simulink model "TRNG_test01"  (R2020a)
settings: Solver=VariableStepAuto  StartTime=0.0  StopTime=100.0  RelTol=1e-3
undefined symbols (not defined in the file): AXI4, Lite
libraries: xbsIndex_r4 x185
settings Model: Creator=ringl  LastModifiedBy=ringl

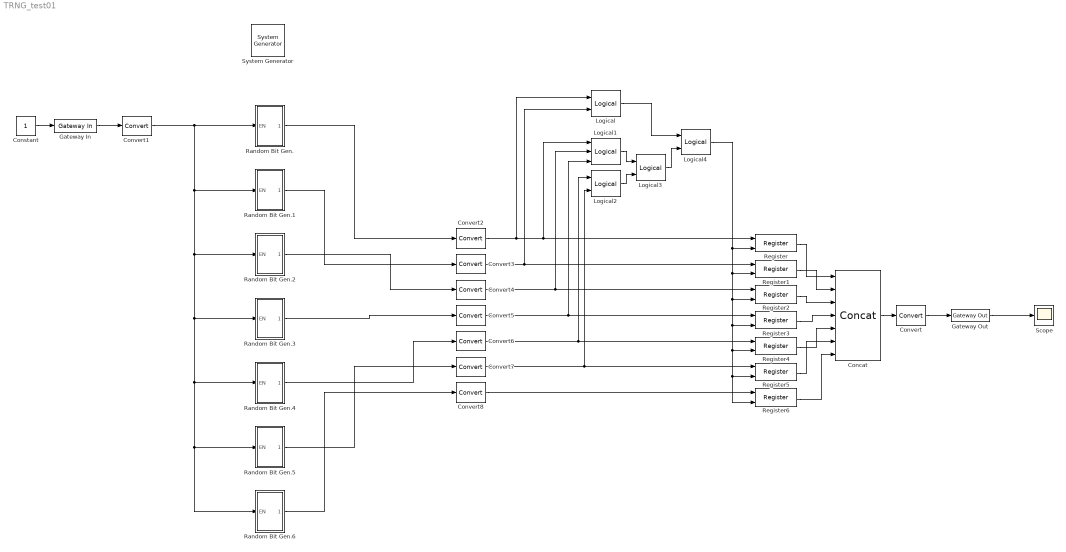
== system TRNG_test01 ==
  " System Generator" : xbsIndex_r4/ System Generator  Tag=genX  xilinxfamily=zynq  part=xc7z020  speed=-1  package=clg400  synthesis_tool=Vivado  clock_wrapper=Clock Enables  directory=./netlist  proj_type=Vivado  Synth_file=Vivado Synthesis Defaults  Impl_file=Vivado Implementation Defaults  testbench=off  simulink_period=1  sysclk_period=10  dcm_input_clock_period=10  incr_netlist=off  trim_vbits=Everywhere in SubSystem  dbl_ovrd=According to Block Masks  core_generation=According to Block Masks  run_coregen=off  deprecated_control=off  eval_field=0  block_type=sysgen
  Concat : xbsIndex_r4/Concat  num_inputs=7  dbl_ovrd=off  block_type=concat
  Constant : Constant
  Convert : xbsIndex_r4/Convert  gui_display_data_type=Fixed-point  arith_type="Signed  (2's comp)"  n_bits=32  bin_pt=0  float_type=Single  exp_bits=8  fraction_bits=24  quantization=Truncate  overflow=Wrap  en=off  latency=1  pipeline=off  dbl_ovrd=off  block_type=convert
  Convert1 : xbsIndex_r4/Convert  gui_display_data_type=Fixed-point  arith_type="Signed  (2's comp)"  n_bits=1  bin_pt=0  float_type=Single  exp_bits=8  fraction_bits=24  quantization=Truncate  overflow=Wrap  en=off  latency=1  pipeline=off  dbl_ovrd=off  block_type=convert
  Convert{2..8} (7 alike) : xbsIndex_r4/Convert  gui_display_data_type=Fixed-point  arith_type=Unsigned  n_bits=1  bin_pt=0  float_type=Single  exp_bits=8  fraction_bits=24  quantization=Truncate  overflow=Wrap  en=off  latency=1  pipeline=off  dbl_ovrd=off  block_type=convert
  Gateway In : xbsIndex_r4/Gateway In  gui_display_data_type=Fixed-point  arith_type="Signed  (2's comp)"  n_bits=32  bin_pt=0  preci_type=Single  exp_width=8  frac_width=24  rows=1  columns=1  quantization="Round  (unbiased: +/- Inf)"  overflow=Saturate  period=1  UseAsADC=off  ADCChannel='1'  interface=AXI4-Lite  automatic_assignment=on  address_offset=hex2dec('00')  intf_name=''  intf_description=''  default_value=0  timing_constraint=None  locs_specified=off  LOCs={}  io_standard={}  inherit_from_input=off  hdl_port=on  dbl_ovrd=off  block_type=gatewayin
  Gateway Out : xbsIndex_r4/Gateway Out  inherit_from_input=off  hdl_port=on  rows=1  columns=1  UseAsDAC=off  DACChannel='1'  interface=AXI4-Lite  automatic_assignment=on  address_offset=hex2dec('00')  intf_name=''  intf_description=''  timing_constraint=None  locs_specified=off  LOCs={}  io_standard={}  block_type=gatewayout
  Logical : xbsIndex_r4/Logical  logical_function=AND  inputs=2  en=off  latency=1  precision=Full  arith_type=Unsigned  n_bits=16  bin_pt=0  align_bp=on  dbl_ovrd=off  block_type=logical
  Logical1 : xbsIndex_r4/Logical  logical_function=AND  inputs=3  en=off  latency=1  precision=Full  arith_type=Unsigned  n_bits=16  bin_pt=0  align_bp=on  dbl_ovrd=off  block_type=logical
  Logical2 : xbsIndex_r4/Logical  logical_function=OR  inputs=2  en=off  latency=1  precision=Full  arith_type=Unsigned  n_bits=16  bin_pt=0  align_bp=on  dbl_ovrd=off  block_type=logical
  Logical3 : xbsIndex_r4/Logical  logical_function=AND  inputs=2  en=off  latency=1  precision=Full  arith_type=Unsigned  n_bits=16  bin_pt=0  align_bp=on  dbl_ovrd=off  block_type=logical
  Logical4 : xbsIndex_r4/Logical  logical_function=NOR  inputs=2  en=off  latency=1  precision=Full  arith_type=Unsigned  n_bits=16  bin_pt=0  align_bp=on  dbl_ovrd=off  block_type=logical
  Random Bit Gen. : Subsystem
  Random Bit Gen.1 : Subsystem
  Random Bit Gen.2 : Subsystem
  Random Bit Gen.3 : Subsystem
  Random Bit Gen.4 : Subsystem
  Random Bit Gen.5 : Subsystem
  Random Bit Gen.6 : Subsystem
  Register{,1..6} (7 alike) : xbsIndex_r4/Register  init=0  rst=off  en=on  dbl_ovrd=off  block_type=register
  Scope : Scope
  wires:
  Constant/1 -> Gateway In/1
  Gateway In/1 -> Convert1/1
  Gateway Out/1 -> Scope/1
  Convert/1 -> Gateway Out/1
  Convert1/1 -> Random Bit Gen.2/1(EN), Random Bit Gen.3/1(EN), Random Bit Gen.4/1(EN), Random Bit Gen.5/1(EN), Random Bit Gen.6/1(EN), Random Bit Gen.1/1(EN), Random Bit Gen./1(EN)
  Random Bit Gen./1(OUT) -> Convert2/1
  Concat/1 -> Convert/1
  Convert2/1 -> Logical/1, Logical1/1, Register/1
  Random Bit Gen.1/1(OUT) -> Convert3/1
  Random Bit Gen.2/1(OUT) -> Convert4/1
  Random Bit Gen.3/1(OUT) -> Convert5/1
  Random Bit Gen.4/1(OUT) -> Convert6/1
  Random Bit Gen.5/1(OUT) -> Convert7/1
  Random Bit Gen.6/1(OUT) -> Convert8/1
  Register3/1 -> Concat/4
  Register4/1 -> Concat/5
  Register5/1 -> Concat/6
  Register6/1 -> Concat/7
  Register2/1 -> Concat/3
  Register1/1 -> Concat/2
  Register/1 -> Concat/1
  Convert3/1 -> Logical/2, Register1/1
  Convert4/1 -> Logical1/2, Register2/1
  Convert5/1 -> Logical1/3, Register3/1
  Convert6/1 -> Logical2/1, Register4/1
  Convert7/1 -> Logical2/2, Register5/1
  Convert8/1 -> Register6/1
  Logical2/1 -> Logical3/2
  Logical1/1 -> Logical3/1
  Logical3/1 -> Logical4/2
  Logical/1 -> Logical4/1
  Logical4/1 -> Register/2, Register1/2, Register2/2, Register3/2, Register4/2, Register5/2, Register6/2

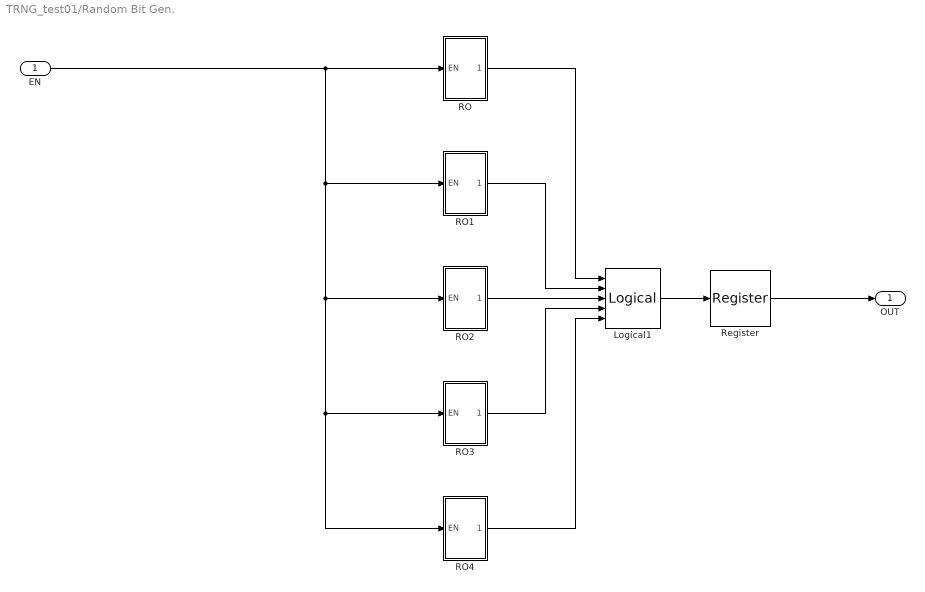
== system TRNG_test01/Random Bit Gen. ==
  EN : Inport
  Logical1 : xbsIndex_r4/Logical  logical_function=XOR  inputs=5  en=off  latency=1  precision=Full  arith_type=Unsigned  n_bits=16  bin_pt=0  align_bp=on  dbl_ovrd=off  block_type=logical
  RO : Subsystem
  RO1 : Subsystem
  RO2 : Subsystem
  RO3 : Subsystem
  RO4 : Subsystem
  Register : xbsIndex_r4/Register  init=0  rst=off  en=off  dbl_ovrd=off  block_type=register
  OUT : Outport
  wires:
  Logical1/1 -> Register/1
  EN/1 -> RO/1(EN), RO1/1(EN), RO2/1(EN), RO4/1(EN), RO3/1(EN)
  RO1/1(OUT) -> Logical1/2
  RO2/1(OUT) -> Logical1/3
  RO/1(OUT) -> Logical1/1
  RO4/1(OUT) -> Logical1/5
  RO3/1(OUT) -> Logical1/4
  Register/1 -> OUT/1

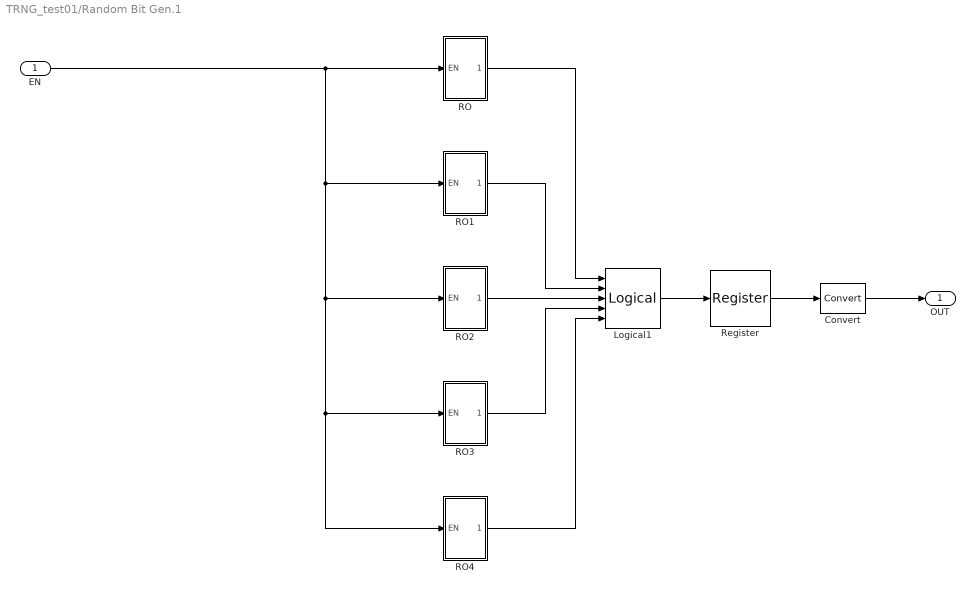
== system TRNG_test01/Random Bit Gen.1 ==
  EN : Inport
  Convert : xbsIndex_r4/Convert  gui_display_data_type=Fixed-point  arith_type="Signed  (2's comp)"  n_bits=1  bin_pt=0  float_type=Single  exp_bits=8  fraction_bits=24  quantization=Truncate  overflow=Wrap  en=off  latency=1  pipeline=off  dbl_ovrd=off  block_type=convert
  Logical1 : xbsIndex_r4/Logical  logical_function=XOR  inputs=5  en=off  latency=1  precision=Full  arith_type=Unsigned  n_bits=16  bin_pt=0  align_bp=on  dbl_ovrd=off  block_type=logical
  RO : Subsystem
  RO1 : Subsystem
  RO2 : Subsystem
  RO3 : Subsystem
  RO4 : Subsystem
  Register : xbsIndex_r4/Register  init=0  rst=off  en=off  dbl_ovrd=off  block_type=register
  OUT : Outport
  wires:
  Logical1/1 -> Register/1
  EN/1 -> RO/1(EN), RO1/1(EN), RO2/1(EN), RO4/1(EN), RO3/1(EN)
  RO1/1(OUT) -> Logical1/2
  RO2/1(OUT) -> Logical1/3
  RO/1(OUT) -> Logical1/1
  RO4/1(OUT) -> Logical1/5
  RO3/1(OUT) -> Logical1/4
  Convert/1 -> OUT/1
  Register/1 -> Convert/1

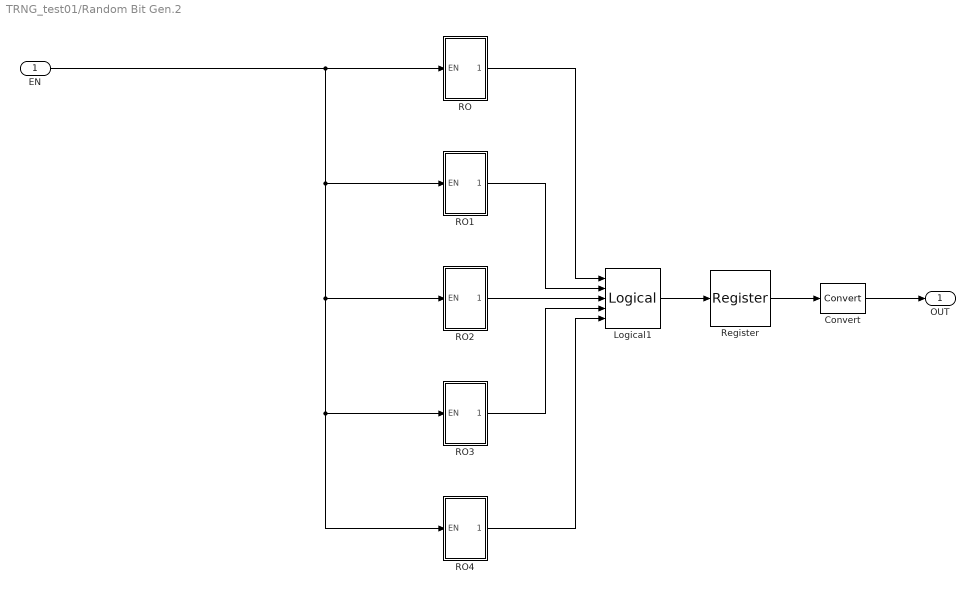
== system TRNG_test01/Random Bit Gen.2 ==
  EN : Inport
  Convert : xbsIndex_r4/Convert  gui_display_data_type=Fixed-point  arith_type="Signed  (2's comp)"  n_bits=1  bin_pt=0  float_type=Single  exp_bits=8  fraction_bits=24  quantization=Truncate  overflow=Wrap  en=off  latency=1  pipeline=off  dbl_ovrd=off  block_type=convert
  Logical1 : xbsIndex_r4/Logical  logical_function=XOR  inputs=5  en=off  latency=1  precision=Full  arith_type=Unsigned  n_bits=16  bin_pt=0  align_bp=on  dbl_ovrd=off  block_type=logical
  RO : Subsystem
  RO1 : Subsystem
  RO2 : Subsystem
  RO3 : Subsystem
  RO4 : Subsystem
  Register : xbsIndex_r4/Register  init=0  rst=off  en=off  dbl_ovrd=off  block_type=register
  OUT : Outport
  wires:
  Logical1/1 -> Register/1
  EN/1 -> RO/1(EN), RO1/1(EN), RO2/1(EN), RO4/1(EN), RO3/1(EN)
  RO1/1(OUT) -> Logical1/2
  RO2/1(OUT) -> Logical1/3
  RO/1(OUT) -> Logical1/1
  RO4/1(OUT) -> Logical1/5
  RO3/1(OUT) -> Logical1/4
  Convert/1 -> OUT/1
  Register/1 -> Convert/1

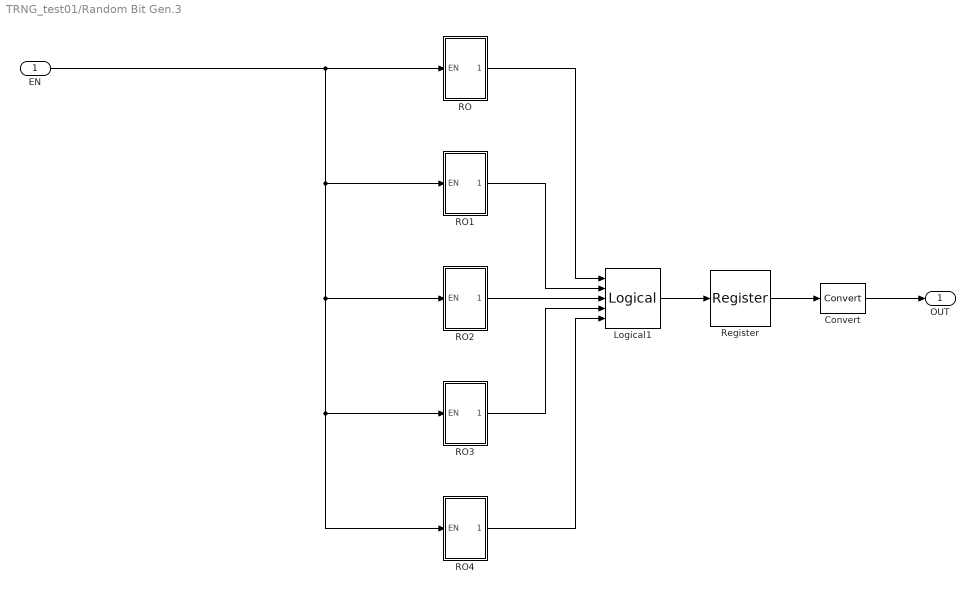
== system TRNG_test01/Random Bit Gen.3 ==
  EN : Inport
  Convert : xbsIndex_r4/Convert  gui_display_data_type=Fixed-point  arith_type="Signed  (2's comp)"  n_bits=1  bin_pt=0  float_type=Single  exp_bits=8  fraction_bits=24  quantization=Truncate  overflow=Wrap  en=off  latency=1  pipeline=off  dbl_ovrd=off  block_type=convert
  Logical1 : xbsIndex_r4/Logical  logical_function=XOR  inputs=5  en=off  latency=1  precision=Full  arith_type=Unsigned  n_bits=16  bin_pt=0  align_bp=on  dbl_ovrd=off  block_type=logical
  RO : Subsystem
  RO1 : Subsystem
  RO2 : Subsystem
  RO3 : Subsystem
  RO4 : Subsystem
  Register : xbsIndex_r4/Register  init=0  rst=off  en=off  dbl_ovrd=off  block_type=register
  OUT : Outport
  wires:
  Logical1/1 -> Register/1
  EN/1 -> RO/1(EN), RO1/1(EN), RO2/1(EN), RO4/1(EN), RO3/1(EN)
  RO1/1(OUT) -> Logical1/2
  RO2/1(OUT) -> Logical1/3
  RO/1(OUT) -> Logical1/1
  RO4/1(OUT) -> Logical1/5
  RO3/1(OUT) -> Logical1/4
  Convert/1 -> OUT/1
  Register/1 -> Convert/1

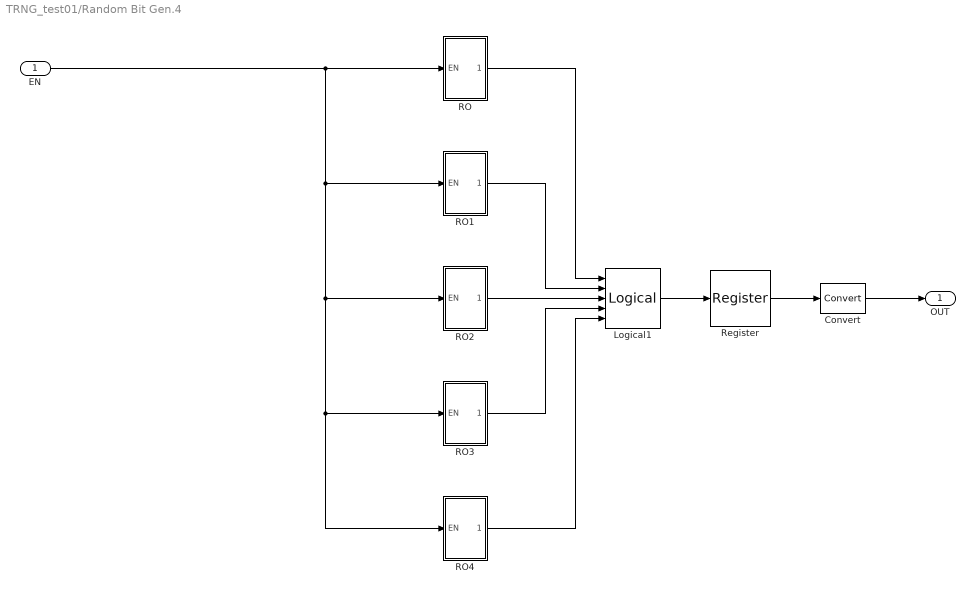
== system TRNG_test01/Random Bit Gen.4 ==
  EN : Inport
  Convert : xbsIndex_r4/Convert  gui_display_data_type=Fixed-point  arith_type="Signed  (2's comp)"  n_bits=1  bin_pt=0  float_type=Single  exp_bits=8  fraction_bits=24  quantization=Truncate  overflow=Wrap  en=off  latency=1  pipeline=off  dbl_ovrd=off  block_type=convert
  Logical1 : xbsIndex_r4/Logical  logical_function=XOR  inputs=5  en=off  latency=1  precision=Full  arith_type=Unsigned  n_bits=16  bin_pt=0  align_bp=on  dbl_ovrd=off  block_type=logical
  RO : Subsystem
  RO1 : Subsystem
  RO2 : Subsystem
  RO3 : Subsystem
  RO4 : Subsystem
  Register : xbsIndex_r4/Register  init=0  rst=off  en=off  dbl_ovrd=off  block_type=register
  OUT : Outport
  wires:
  Logical1/1 -> Register/1
  EN/1 -> RO/1(EN), RO1/1(EN), RO2/1(EN), RO4/1(EN), RO3/1(EN)
  RO1/1(OUT) -> Logical1/2
  RO2/1(OUT) -> Logical1/3
  RO/1(OUT) -> Logical1/1
  RO4/1(OUT) -> Logical1/5
  RO3/1(OUT) -> Logical1/4
  Convert/1 -> OUT/1
  Register/1 -> Convert/1

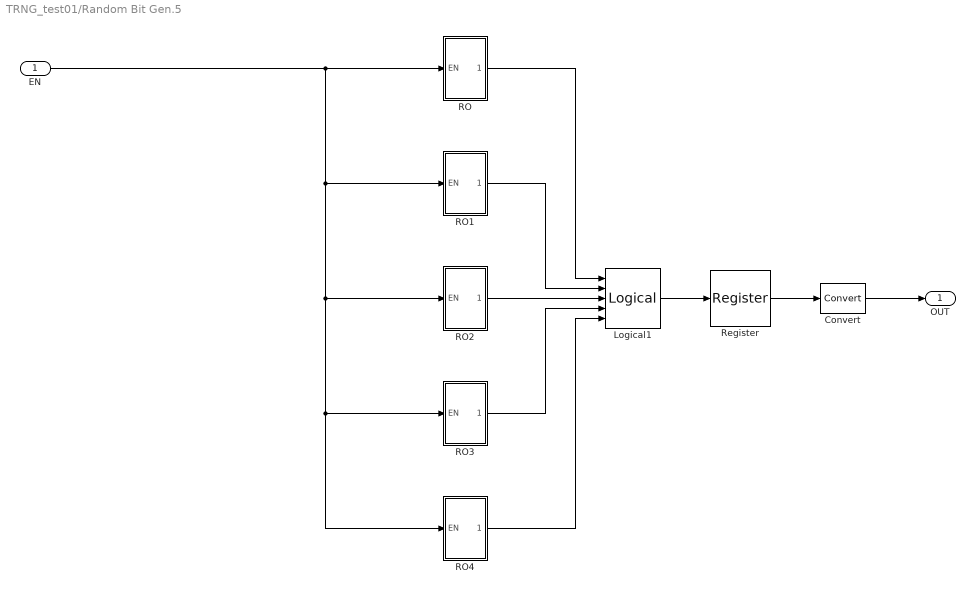
== system TRNG_test01/Random Bit Gen.5 ==
  EN : Inport
  Convert : xbsIndex_r4/Convert  gui_display_data_type=Fixed-point  arith_type="Signed  (2's comp)"  n_bits=1  bin_pt=0  float_type=Single  exp_bits=8  fraction_bits=24  quantization=Truncate  overflow=Wrap  en=off  latency=1  pipeline=off  dbl_ovrd=off  block_type=convert
  Logical1 : xbsIndex_r4/Logical  logical_function=XOR  inputs=5  en=off  latency=1  precision=Full  arith_type=Unsigned  n_bits=16  bin_pt=0  align_bp=on  dbl_ovrd=off  block_type=logical
  RO : Subsystem
  RO1 : Subsystem
  RO2 : Subsystem
  RO3 : Subsystem
  RO4 : Subsystem
  Register : xbsIndex_r4/Register  init=0  rst=off  en=off  dbl_ovrd=off  block_type=register
  OUT : Outport
  wires:
  Logical1/1 -> Register/1
  EN/1 -> RO/1(EN), RO1/1(EN), RO2/1(EN), RO4/1(EN), RO3/1(EN)
  RO1/1(OUT) -> Logical1/2
  RO2/1(OUT) -> Logical1/3
  RO/1(OUT) -> Logical1/1
  RO4/1(OUT) -> Logical1/5
  RO3/1(OUT) -> Logical1/4
  Convert/1 -> OUT/1
  Register/1 -> Convert/1

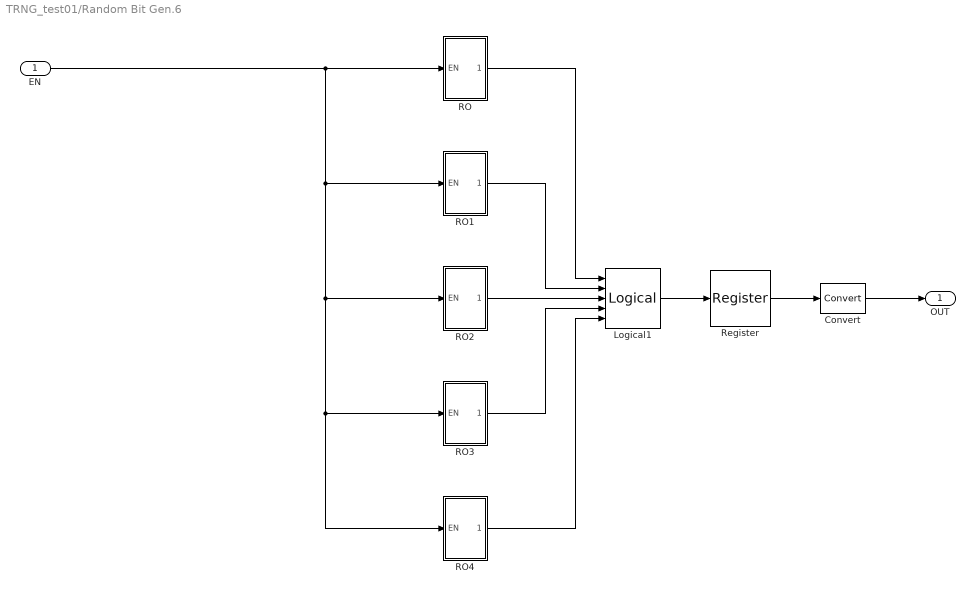
== system TRNG_test01/Random Bit Gen.6 ==
  EN : Inport
  Convert : xbsIndex_r4/Convert  gui_display_data_type=Fixed-point  arith_type="Signed  (2's comp)"  n_bits=1  bin_pt=0  float_type=Single  exp_bits=8  fraction_bits=24  quantization=Truncate  overflow=Wrap  en=off  latency=1  pipeline=off  dbl_ovrd=off  block_type=convert
  Logical1 : xbsIndex_r4/Logical  logical_function=XOR  inputs=5  en=off  latency=1  precision=Full  arith_type=Unsigned  n_bits=16  bin_pt=0  align_bp=on  dbl_ovrd=off  block_type=logical
  RO : Subsystem
  RO1 : Subsystem
  RO2 : Subsystem
  RO3 : Subsystem
  RO4 : Subsystem
  Register : xbsIndex_r4/Register  init=0  rst=off  en=off  dbl_ovrd=off  block_type=register
  OUT : Outport
  wires:
  Logical1/1 -> Register/1
  EN/1 -> RO/1(EN), RO1/1(EN), RO2/1(EN), RO4/1(EN), RO3/1(EN)
  RO1/1(OUT) -> Logical1/2
  RO2/1(OUT) -> Logical1/3
  RO/1(OUT) -> Logical1/1
  RO4/1(OUT) -> Logical1/5
  RO3/1(OUT) -> Logical1/4
  Convert/1 -> OUT/1
  Register/1 -> Convert/1

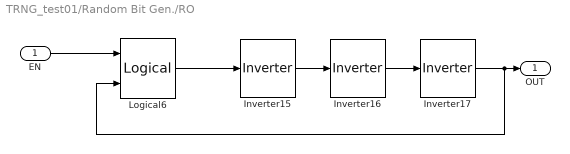
== system TRNG_test01/Random Bit Gen./RO ==
  EN : Inport
  Inverter15 : xbsIndex_r4/Inverter  en=off  latency=1  dbl_ovrd=off  block_type=inv
  Inverter16 : xbsIndex_r4/Inverter  en=off  latency=1  dbl_ovrd=off  block_type=inv
  Inverter17 : xbsIndex_r4/Inverter  en=off  latency=1  dbl_ovrd=off  block_type=inv
  Logical6 : xbsIndex_r4/Logical  logical_function=AND  inputs=2  en=off  latency=1  precision=Full  arith_type=Unsigned  n_bits=16  bin_pt=0  align_bp=on  dbl_ovrd=off  block_type=logical
  OUT : Outport
  wires:
  Logical6/1 -> Inverter15/1
  Inverter17/1 -> OUT/1, Logical6/2
  Inverter16/1 -> Inverter17/1
  EN/1 -> Logical6/1
  Inverter15/1 -> Inverter16/1

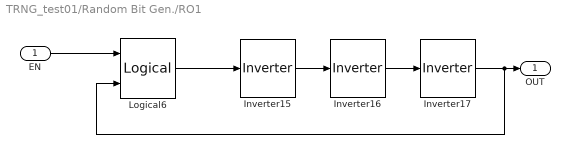
== system TRNG_test01/Random Bit Gen./RO1 ==
  EN : Inport
  Inverter15 : xbsIndex_r4/Inverter  en=off  latency=1  dbl_ovrd=off  block_type=inv
  Inverter16 : xbsIndex_r4/Inverter  en=off  latency=1  dbl_ovrd=off  block_type=inv
  Inverter17 : xbsIndex_r4/Inverter  en=off  latency=1  dbl_ovrd=off  block_type=inv
  Logical6 : xbsIndex_r4/Logical  logical_function=AND  inputs=2  en=off  latency=1  precision=Full  arith_type=Unsigned  n_bits=16  bin_pt=0  align_bp=on  dbl_ovrd=off  block_type=logical
  OUT : Outport
  wires:
  Logical6/1 -> Inverter15/1
  Inverter17/1 -> OUT/1, Logical6/2
  Inverter16/1 -> Inverter17/1
  EN/1 -> Logical6/1
  Inverter15/1 -> Inverter16/1

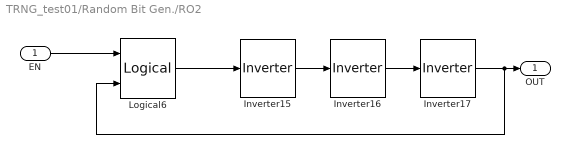
== system TRNG_test01/Random Bit Gen./RO2 ==
  EN : Inport
  Inverter15 : xbsIndex_r4/Inverter  en=off  latency=1  dbl_ovrd=off  block_type=inv
  Inverter16 : xbsIndex_r4/Inverter  en=off  latency=1  dbl_ovrd=off  block_type=inv
  Inverter17 : xbsIndex_r4/Inverter  en=off  latency=1  dbl_ovrd=off  block_type=inv
  Logical6 : xbsIndex_r4/Logical  logical_function=AND  inputs=2  en=off  latency=1  precision=Full  arith_type=Unsigned  n_bits=16  bin_pt=0  align_bp=on  dbl_ovrd=off  block_type=logical
  OUT : Outport
  wires:
  Logical6/1 -> Inverter15/1
  Inverter17/1 -> OUT/1, Logical6/2
  Inverter16/1 -> Inverter17/1
  EN/1 -> Logical6/1
  Inverter15/1 -> Inverter16/1

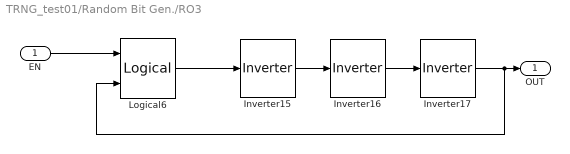
== system TRNG_test01/Random Bit Gen./RO3 ==
  EN : Inport
  Inverter15 : xbsIndex_r4/Inverter  en=off  latency=1  dbl_ovrd=off  block_type=inv
  Inverter16 : xbsIndex_r4/Inverter  en=off  latency=1  dbl_ovrd=off  block_type=inv
  Inverter17 : xbsIndex_r4/Inverter  en=off  latency=1  dbl_ovrd=off  block_type=inv
  Logical6 : xbsIndex_r4/Logical  logical_function=AND  inputs=2  en=off  latency=1  precision=Full  arith_type=Unsigned  n_bits=16  bin_pt=0  align_bp=on  dbl_ovrd=off  block_type=logical
  OUT : Outport
  wires:
  Logical6/1 -> Inverter15/1
  Inverter17/1 -> OUT/1, Logical6/2
  Inverter16/1 -> Inverter17/1
  EN/1 -> Logical6/1
  Inverter15/1 -> Inverter16/1

== system TRNG_test01/Random Bit Gen./RO4 ==
  EN : Inport
  Inverter15 : xbsIndex_r4/Inverter  en=off  latency=1  dbl_ovrd=off  block_type=inv
  Inverter16 : xbsIndex_r4/Inverter  en=off  latency=1  dbl_ovrd=off  block_type=inv
  Inverter17 : xbsIndex_r4/Inverter  en=off  latency=1  dbl_ovrd=off  block_type=inv
  Logical6 : xbsIndex_r4/Logical  logical_function=AND  inputs=2  en=off  latency=1  precision=Full  arith_type=Unsigned  n_bits=16  bin_pt=0  align_bp=on  dbl_ovrd=off  block_type=logical
  OUT : Outport
  wires:
  Logical6/1 -> Inverter15/1
  Inverter17/1 -> OUT/1, Logical6/2
  Inverter16/1 -> Inverter17/1
  EN/1 -> Logical6/1
  Inverter15/1 -> Inverter16/1

== system TRNG_test01/Random Bit Gen.1/RO ==
  EN : Inport
  Inverter15 : xbsIndex_r4/Inverter  en=off  latency=1  dbl_ovrd=off  block_type=inv
  Inverter16 : xbsIndex_r4/Inverter  en=off  latency=1  dbl_ovrd=off  block_type=inv
  Inverter17 : xbsIndex_r4/Inverter  en=off  latency=1  dbl_ovrd=off  block_type=inv
  Logical6 : xbsIndex_r4/Logical  logical_function=AND  inputs=2  en=off  latency=1  precision=Full  arith_type=Unsigned  n_bits=16  bin_pt=0  align_bp=on  dbl_ovrd=off  block_type=logical
  OUT : Outport
  wires:
  Logical6/1 -> Inverter15/1
  Inverter17/1 -> OUT/1, Logical6/2
  Inverter16/1 -> Inverter17/1
  EN/1 -> Logical6/1
  Inverter15/1 -> Inverter16/1

== system TRNG_test01/Random Bit Gen.1/RO1 ==
  EN : Inport
  Inverter15 : xbsIndex_r4/Inverter  en=off  latency=1  dbl_ovrd=off  block_type=inv
  Inverter16 : xbsIndex_r4/Inverter  en=off  latency=1  dbl_ovrd=off  block_type=inv
  Inverter17 : xbsIndex_r4/Inverter  en=off  latency=1  dbl_ovrd=off  block_type=inv
  Logical6 : xbsIndex_r4/Logical  logical_function=AND  inputs=2  en=off  latency=1  precision=Full  arith_type=Unsigned  n_bits=16  bin_pt=0  align_bp=on  dbl_ovrd=off  block_type=logical
  OUT : Outport
  wires:
  Logical6/1 -> Inverter15/1
  Inverter17/1 -> OUT/1, Logical6/2
  Inverter16/1 -> Inverter17/1
  EN/1 -> Logical6/1
  Inverter15/1 -> Inverter16/1

== system TRNG_test01/Random Bit Gen.1/RO2 ==
  EN : Inport
  Inverter15 : xbsIndex_r4/Inverter  en=off  latency=1  dbl_ovrd=off  block_type=inv
  Inverter16 : xbsIndex_r4/Inverter  en=off  latency=1  dbl_ovrd=off  block_type=inv
  Inverter17 : xbsIndex_r4/Inverter  en=off  latency=1  dbl_ovrd=off  block_type=inv
  Logical6 : xbsIndex_r4/Logical  logical_function=AND  inputs=2  en=off  latency=1  precision=Full  arith_type=Unsigned  n_bits=16  bin_pt=0  align_bp=on  dbl_ovrd=off  block_type=logical
  OUT : Outport
  wires:
  Logical6/1 -> Inverter15/1
  Inverter17/1 -> OUT/1, Logical6/2
  Inverter16/1 -> Inverter17/1
  EN/1 -> Logical6/1
  Inverter15/1 -> Inverter16/1

== system TRNG_test01/Random Bit Gen.1/RO3 ==
  EN : Inport
  Inverter15 : xbsIndex_r4/Inverter  en=off  latency=1  dbl_ovrd=off  block_type=inv
  Inverter16 : xbsIndex_r4/Inverter  en=off  latency=1  dbl_ovrd=off  block_type=inv
  Inverter17 : xbsIndex_r4/Inverter  en=off  latency=1  dbl_ovrd=off  block_type=inv
  Logical6 : xbsIndex_r4/Logical  logical_function=AND  inputs=2  en=off  latency=1  precision=Full  arith_type=Unsigned  n_bits=16  bin_pt=0  align_bp=on  dbl_ovrd=off  block_type=logical
  OUT : Outport
  wires:
  Logical6/1 -> Inverter15/1
  Inverter17/1 -> OUT/1, Logical6/2
  Inverter16/1 -> Inverter17/1
  EN/1 -> Logical6/1
  Inverter15/1 -> Inverter16/1

== system TRNG_test01/Random Bit Gen.1/RO4 ==
  EN : Inport
  Inverter15 : xbsIndex_r4/Inverter  en=off  latency=1  dbl_ovrd=off  block_type=inv
  Inverter16 : xbsIndex_r4/Inverter  en=off  latency=1  dbl_ovrd=off  block_type=inv
  Inverter17 : xbsIndex_r4/Inverter  en=off  latency=1  dbl_ovrd=off  block_type=inv
  Logical6 : xbsIndex_r4/Logical  logical_function=AND  inputs=2  en=off  latency=1  precision=Full  arith_type=Unsigned  n_bits=16  bin_pt=0  align_bp=on  dbl_ovrd=off  block_type=logical
  OUT : Outport
  wires:
  Logical6/1 -> Inverter15/1
  Inverter17/1 -> OUT/1, Logical6/2
  Inverter16/1 -> Inverter17/1
  EN/1 -> Logical6/1
  Inverter15/1 -> Inverter16/1

== system TRNG_test01/Random Bit Gen.2/RO ==
  EN : Inport
  Inverter15 : xbsIndex_r4/Inverter  en=off  latency=1  dbl_ovrd=off  block_type=inv
  Inverter16 : xbsIndex_r4/Inverter  en=off  latency=1  dbl_ovrd=off  block_type=inv
  Inverter17 : xbsIndex_r4/Inverter  en=off  latency=1  dbl_ovrd=off  block_type=inv
  Logical6 : xbsIndex_r4/Logical  logical_function=AND  inputs=2  en=off  latency=1  precision=Full  arith_type=Unsigned  n_bits=16  bin_pt=0  align_bp=on  dbl_ovrd=off  block_type=logical
  OUT : Outport
  wires:
  Logical6/1 -> Inverter15/1
  Inverter17/1 -> OUT/1, Logical6/2
  Inverter16/1 -> Inverter17/1
  EN/1 -> Logical6/1
  Inverter15/1 -> Inverter16/1

== system TRNG_test01/Random Bit Gen.2/RO1 ==
  EN : Inport
  Inverter15 : xbsIndex_r4/Inverter  en=off  latency=1  dbl_ovrd=off  block_type=inv
  Inverter16 : xbsIndex_r4/Inverter  en=off  latency=1  dbl_ovrd=off  block_type=inv
  Inverter17 : xbsIndex_r4/Inverter  en=off  latency=1  dbl_ovrd=off  block_type=inv
  Logical6 : xbsIndex_r4/Logical  logical_function=AND  inputs=2  en=off  latency=1  precision=Full  arith_type=Unsigned  n_bits=16  bin_pt=0  align_bp=on  dbl_ovrd=off  block_type=logical
  OUT : Outport
  wires:
  Logical6/1 -> Inverter15/1
  Inverter17/1 -> OUT/1, Logical6/2
  Inverter16/1 -> Inverter17/1
  EN/1 -> Logical6/1
  Inverter15/1 -> Inverter16/1

== system TRNG_test01/Random Bit Gen.2/RO2 ==
  EN : Inport
  Inverter15 : xbsIndex_r4/Inverter  en=off  latency=1  dbl_ovrd=off  block_type=inv
  Inverter16 : xbsIndex_r4/Inverter  en=off  latency=1  dbl_ovrd=off  block_type=inv
  Inverter17 : xbsIndex_r4/Inverter  en=off  latency=1  dbl_ovrd=off  block_type=inv
  Logical6 : xbsIndex_r4/Logical  logical_function=AND  inputs=2  en=off  latency=1  precision=Full  arith_type=Unsigned  n_bits=16  bin_pt=0  align_bp=on  dbl_ovrd=off  block_type=logical
  OUT : Outport
  wires:
  Logical6/1 -> Inverter15/1
  Inverter17/1 -> OUT/1, Logical6/2
  Inverter16/1 -> Inverter17/1
  EN/1 -> Logical6/1
  Inverter15/1 -> Inverter16/1

== system TRNG_test01/Random Bit Gen.2/RO3 ==
  EN : Inport
  Inverter15 : xbsIndex_r4/Inverter  en=off  latency=1  dbl_ovrd=off  block_type=inv
  Inverter16 : xbsIndex_r4/Inverter  en=off  latency=1  dbl_ovrd=off  block_type=inv
  Inverter17 : xbsIndex_r4/Inverter  en=off  latency=1  dbl_ovrd=off  block_type=inv
  Logical6 : xbsIndex_r4/Logical  logical_function=AND  inputs=2  en=off  latency=1  precision=Full  arith_type=Unsigned  n_bits=16  bin_pt=0  align_bp=on  dbl_ovrd=off  block_type=logical
  OUT : Outport
  wires:
  Logical6/1 -> Inverter15/1
  Inverter17/1 -> OUT/1, Logical6/2
  Inverter16/1 -> Inverter17/1
  EN/1 -> Logical6/1
  Inverter15/1 -> Inverter16/1

== system TRNG_test01/Random Bit Gen.2/RO4 ==
  EN : Inport
  Inverter15 : xbsIndex_r4/Inverter  en=off  latency=1  dbl_ovrd=off  block_type=inv
  Inverter16 : xbsIndex_r4/Inverter  en=off  latency=1  dbl_ovrd=off  block_type=inv
  Inverter17 : xbsIndex_r4/Inverter  en=off  latency=1  dbl_ovrd=off  block_type=inv
  Logical6 : xbsIndex_r4/Logical  logical_function=AND  inputs=2  en=off  latency=1  precision=Full  arith_type=Unsigned  n_bits=16  bin_pt=0  align_bp=on  dbl_ovrd=off  block_type=logical
  OUT : Outport
  wires:
  Logical6/1 -> Inverter15/1
  Inverter17/1 -> OUT/1, Logical6/2
  Inverter16/1 -> Inverter17/1
  EN/1 -> Logical6/1
  Inverter15/1 -> Inverter16/1

== system TRNG_test01/Random Bit Gen.3/RO ==
  EN : Inport
  Inverter15 : xbsIndex_r4/Inverter  en=off  latency=1  dbl_ovrd=off  block_type=inv
  Inverter16 : xbsIndex_r4/Inverter  en=off  latency=1  dbl_ovrd=off  block_type=inv
  Inverter17 : xbsIndex_r4/Inverter  en=off  latency=1  dbl_ovrd=off  block_type=inv
  Logical6 : xbsIndex_r4/Logical  logical_function=AND  inputs=2  en=off  latency=1  precision=Full  arith_type=Unsigned  n_bits=16  bin_pt=0  align_bp=on  dbl_ovrd=off  block_type=logical
  OUT : Outport
  wires:
  Logical6/1 -> Inverter15/1
  Inverter17/1 -> OUT/1, Logical6/2
  Inverter16/1 -> Inverter17/1
  EN/1 -> Logical6/1
  Inverter15/1 -> Inverter16/1

== system TRNG_test01/Random Bit Gen.3/RO1 ==
  EN : Inport
  Inverter15 : xbsIndex_r4/Inverter  en=off  latency=1  dbl_ovrd=off  block_type=inv
  Inverter16 : xbsIndex_r4/Inverter  en=off  latency=1  dbl_ovrd=off  block_type=inv
  Inverter17 : xbsIndex_r4/Inverter  en=off  latency=1  dbl_ovrd=off  block_type=inv
  Logical6 : xbsIndex_r4/Logical  logical_function=AND  inputs=2  en=off  latency=1  precision=Full  arith_type=Unsigned  n_bits=16  bin_pt=0  align_bp=on  dbl_ovrd=off  block_type=logical
  OUT : Outport
  wires:
  Logical6/1 -> Inverter15/1
  Inverter17/1 -> OUT/1, Logical6/2
  Inverter16/1 -> Inverter17/1
  EN/1 -> Logical6/1
  Inverter15/1 -> Inverter16/1

== system TRNG_test01/Random Bit Gen.3/RO2 ==
  EN : Inport
  Inverter15 : xbsIndex_r4/Inverter  en=off  latency=1  dbl_ovrd=off  block_type=inv
  Inverter16 : xbsIndex_r4/Inverter  en=off  latency=1  dbl_ovrd=off  block_type=inv
  Inverter17 : xbsIndex_r4/Inverter  en=off  latency=1  dbl_ovrd=off  block_type=inv
  Logical6 : xbsIndex_r4/Logical  logical_function=AND  inputs=2  en=off  latency=1  precision=Full  arith_type=Unsigned  n_bits=16  bin_pt=0  align_bp=on  dbl_ovrd=off  block_type=logical
  OUT : Outport
  wires:
  Logical6/1 -> Inverter15/1
  Inverter17/1 -> OUT/1, Logical6/2
  Inverter16/1 -> Inverter17/1
  EN/1 -> Logical6/1
  Inverter15/1 -> Inverter16/1

== system TRNG_test01/Random Bit Gen.3/RO3 ==
  EN : Inport
  Inverter15 : xbsIndex_r4/Inverter  en=off  latency=1  dbl_ovrd=off  block_type=inv
  Inverter16 : xbsIndex_r4/Inverter  en=off  latency=1  dbl_ovrd=off  block_type=inv
  Inverter17 : xbsIndex_r4/Inverter  en=off  latency=1  dbl_ovrd=off  block_type=inv
  Logical6 : xbsIndex_r4/Logical  logical_function=AND  inputs=2  en=off  latency=1  precision=Full  arith_type=Unsigned  n_bits=16  bin_pt=0  align_bp=on  dbl_ovrd=off  block_type=logical
  OUT : Outport
  wires:
  Logical6/1 -> Inverter15/1
  Inverter17/1 -> OUT/1, Logical6/2
  Inverter16/1 -> Inverter17/1
  EN/1 -> Logical6/1
  Inverter15/1 -> Inverter16/1

== system TRNG_test01/Random Bit Gen.3/RO4 ==
  EN : Inport
  Inverter15 : xbsIndex_r4/Inverter  en=off  latency=1  dbl_ovrd=off  block_type=inv
  Inverter16 : xbsIndex_r4/Inverter  en=off  latency=1  dbl_ovrd=off  block_type=inv
  Inverter17 : xbsIndex_r4/Inverter  en=off  latency=1  dbl_ovrd=off  block_type=inv
  Logical6 : xbsIndex_r4/Logical  logical_function=AND  inputs=2  en=off  latency=1  precision=Full  arith_type=Unsigned  n_bits=16  bin_pt=0  align_bp=on  dbl_ovrd=off  block_type=logical
  OUT : Outport
  wires:
  Logical6/1 -> Inverter15/1
  Inverter17/1 -> OUT/1, Logical6/2
  Inverter16/1 -> Inverter17/1
  EN/1 -> Logical6/1
  Inverter15/1 -> Inverter16/1

== system TRNG_test01/Random Bit Gen.4/RO ==
  EN : Inport
  Inverter15 : xbsIndex_r4/Inverter  en=off  latency=1  dbl_ovrd=off  block_type=inv
  Inverter16 : xbsIndex_r4/Inverter  en=off  latency=1  dbl_ovrd=off  block_type=inv
  Inverter17 : xbsIndex_r4/Inverter  en=off  latency=1  dbl_ovrd=off  block_type=inv
  Logical6 : xbsIndex_r4/Logical  logical_function=AND  inputs=2  en=off  latency=1  precision=Full  arith_type=Unsigned  n_bits=16  bin_pt=0  align_bp=on  dbl_ovrd=off  block_type=logical
  OUT : Outport
  wires:
  Logical6/1 -> Inverter15/1
  Inverter17/1 -> OUT/1, Logical6/2
  Inverter16/1 -> Inverter17/1
  EN/1 -> Logical6/1
  Inverter15/1 -> Inverter16/1

== system TRNG_test01/Random Bit Gen.4/RO1 ==
  EN : Inport
  Inverter15 : xbsIndex_r4/Inverter  en=off  latency=1  dbl_ovrd=off  block_type=inv
  Inverter16 : xbsIndex_r4/Inverter  en=off  latency=1  dbl_ovrd=off  block_type=inv
  Inverter17 : xbsIndex_r4/Inverter  en=off  latency=1  dbl_ovrd=off  block_type=inv
  Logical6 : xbsIndex_r4/Logical  logical_function=AND  inputs=2  en=off  latency=1  precision=Full  arith_type=Unsigned  n_bits=16  bin_pt=0  align_bp=on  dbl_ovrd=off  block_type=logical
  OUT : Outport
  wires:
  Logical6/1 -> Inverter15/1
  Inverter17/1 -> OUT/1, Logical6/2
  Inverter16/1 -> Inverter17/1
  EN/1 -> Logical6/1
  Inverter15/1 -> Inverter16/1

== system TRNG_test01/Random Bit Gen.4/RO2 ==
  EN : Inport
  Inverter15 : xbsIndex_r4/Inverter  en=off  latency=1  dbl_ovrd=off  block_type=inv
  Inverter16 : xbsIndex_r4/Inverter  en=off  latency=1  dbl_ovrd=off  block_type=inv
  Inverter17 : xbsIndex_r4/Inverter  en=off  latency=1  dbl_ovrd=off  block_type=inv
  Logical6 : xbsIndex_r4/Logical  logical_function=AND  inputs=2  en=off  latency=1  precision=Full  arith_type=Unsigned  n_bits=16  bin_pt=0  align_bp=on  dbl_ovrd=off  block_type=logical
  OUT : Outport
  wires:
  Logical6/1 -> Inverter15/1
  Inverter17/1 -> OUT/1, Logical6/2
  Inverter16/1 -> Inverter17/1
  EN/1 -> Logical6/1
  Inverter15/1 -> Inverter16/1

== system TRNG_test01/Random Bit Gen.4/RO3 ==
  EN : Inport
  Inverter15 : xbsIndex_r4/Inverter  en=off  latency=1  dbl_ovrd=off  block_type=inv
  Inverter16 : xbsIndex_r4/Inverter  en=off  latency=1  dbl_ovrd=off  block_type=inv
  Inverter17 : xbsIndex_r4/Inverter  en=off  latency=1  dbl_ovrd=off  block_type=inv
  Logical6 : xbsIndex_r4/Logical  logical_function=AND  inputs=2  en=off  latency=1  precision=Full  arith_type=Unsigned  n_bits=16  bin_pt=0  align_bp=on  dbl_ovrd=off  block_type=logical
  OUT : Outport
  wires:
  Logical6/1 -> Inverter15/1
  Inverter17/1 -> OUT/1, Logical6/2
  Inverter16/1 -> Inverter17/1
  EN/1 -> Logical6/1
  Inverter15/1 -> Inverter16/1

== system TRNG_test01/Random Bit Gen.4/RO4 ==
  EN : Inport
  Inverter15 : xbsIndex_r4/Inverter  en=off  latency=1  dbl_ovrd=off  block_type=inv
  Inverter16 : xbsIndex_r4/Inverter  en=off  latency=1  dbl_ovrd=off  block_type=inv
  Inverter17 : xbsIndex_r4/Inverter  en=off  latency=1  dbl_ovrd=off  block_type=inv
  Logical6 : xbsIndex_r4/Logical  logical_function=AND  inputs=2  en=off  latency=1  precision=Full  arith_type=Unsigned  n_bits=16  bin_pt=0  align_bp=on  dbl_ovrd=off  block_type=logical
  OUT : Outport
  wires:
  Logical6/1 -> Inverter15/1
  Inverter17/1 -> OUT/1, Logical6/2
  Inverter16/1 -> Inverter17/1
  EN/1 -> Logical6/1
  Inverter15/1 -> Inverter16/1

== system TRNG_test01/Random Bit Gen.5/RO ==
  EN : Inport
  Inverter15 : xbsIndex_r4/Inverter  en=off  latency=1  dbl_ovrd=off  block_type=inv
  Inverter16 : xbsIndex_r4/Inverter  en=off  latency=1  dbl_ovrd=off  block_type=inv
  Inverter17 : xbsIndex_r4/Inverter  en=off  latency=1  dbl_ovrd=off  block_type=inv
  Logical6 : xbsIndex_r4/Logical  logical_function=AND  inputs=2  en=off  latency=1  precision=Full  arith_type=Unsigned  n_bits=16  bin_pt=0  align_bp=on  dbl_ovrd=off  block_type=logical
  OUT : Outport
  wires:
  Logical6/1 -> Inverter15/1
  Inverter17/1 -> OUT/1, Logical6/2
  Inverter16/1 -> Inverter17/1
  EN/1 -> Logical6/1
  Inverter15/1 -> Inverter16/1

== system TRNG_test01/Random Bit Gen.5/RO1 ==
  EN : Inport
  Inverter15 : xbsIndex_r4/Inverter  en=off  latency=1  dbl_ovrd=off  block_type=inv
  Inverter16 : xbsIndex_r4/Inverter  en=off  latency=1  dbl_ovrd=off  block_type=inv
  Inverter17 : xbsIndex_r4/Inverter  en=off  latency=1  dbl_ovrd=off  block_type=inv
  Logical6 : xbsIndex_r4/Logical  logical_function=AND  inputs=2  en=off  latency=1  precision=Full  arith_type=Unsigned  n_bits=16  bin_pt=0  align_bp=on  dbl_ovrd=off  block_type=logical
  OUT : Outport
  wires:
  Logical6/1 -> Inverter15/1
  Inverter17/1 -> OUT/1, Logical6/2
  Inverter16/1 -> Inverter17/1
  EN/1 -> Logical6/1
  Inverter15/1 -> Inverter16/1

== system TRNG_test01/Random Bit Gen.5/RO2 ==
  EN : Inport
  Inverter15 : xbsIndex_r4/Inverter  en=off  latency=1  dbl_ovrd=off  block_type=inv
  Inverter16 : xbsIndex_r4/Inverter  en=off  latency=1  dbl_ovrd=off  block_type=inv
  Inverter17 : xbsIndex_r4/Inverter  en=off  latency=1  dbl_ovrd=off  block_type=inv
  Logical6 : xbsIndex_r4/Logical  logical_function=AND  inputs=2  en=off  latency=1  precision=Full  arith_type=Unsigned  n_bits=16  bin_pt=0  align_bp=on  dbl_ovrd=off  block_type=logical
  OUT : Outport
  wires:
  Logical6/1 -> Inverter15/1
  Inverter17/1 -> OUT/1, Logical6/2
  Inverter16/1 -> Inverter17/1
  EN/1 -> Logical6/1
  Inverter15/1 -> Inverter16/1

== system TRNG_test01/Random Bit Gen.5/RO3 ==
  EN : Inport
  Inverter15 : xbsIndex_r4/Inverter  en=off  latency=1  dbl_ovrd=off  block_type=inv
  Inverter16 : xbsIndex_r4/Inverter  en=off  latency=1  dbl_ovrd=off  block_type=inv
  Inverter17 : xbsIndex_r4/Inverter  en=off  latency=1  dbl_ovrd=off  block_type=inv
  Logical6 : xbsIndex_r4/Logical  logical_function=AND  inputs=2  en=off  latency=1  precision=Full  arith_type=Unsigned  n_bits=16  bin_pt=0  align_bp=on  dbl_ovrd=off  block_type=logical
  OUT : Outport
  wires:
  Logical6/1 -> Inverter15/1
  Inverter17/1 -> OUT/1, Logical6/2
  Inverter16/1 -> Inverter17/1
  EN/1 -> Logical6/1
  Inverter15/1 -> Inverter16/1

== system TRNG_test01/Random Bit Gen.5/RO4 ==
  EN : Inport
  Inverter15 : xbsIndex_r4/Inverter  en=off  latency=1  dbl_ovrd=off  block_type=inv
  Inverter16 : xbsIndex_r4/Inverter  en=off  latency=1  dbl_ovrd=off  block_type=inv
  Inverter17 : xbsIndex_r4/Inverter  en=off  latency=1  dbl_ovrd=off  block_type=inv
  Logical6 : xbsIndex_r4/Logical  logical_function=AND  inputs=2  en=off  latency=1  precision=Full  arith_type=Unsigned  n_bits=16  bin_pt=0  align_bp=on  dbl_ovrd=off  block_type=logical
  OUT : Outport
  wires:
  Logical6/1 -> Inverter15/1
  Inverter17/1 -> OUT/1, Logical6/2
  Inverter16/1 -> Inverter17/1
  EN/1 -> Logical6/1
  Inverter15/1 -> Inverter16/1

== system TRNG_test01/Random Bit Gen.6/RO ==
  EN : Inport
  Inverter15 : xbsIndex_r4/Inverter  en=off  latency=1  dbl_ovrd=off  block_type=inv
  Inverter16 : xbsIndex_r4/Inverter  en=off  latency=1  dbl_ovrd=off  block_type=inv
  Inverter17 : xbsIndex_r4/Inverter  en=off  latency=1  dbl_ovrd=off  block_type=inv
  Logical6 : xbsIndex_r4/Logical  logical_function=AND  inputs=2  en=off  latency=1  precision=Full  arith_type=Unsigned  n_bits=16  bin_pt=0  align_bp=on  dbl_ovrd=off  block_type=logical
  OUT : Outport
  wires:
  Logical6/1 -> Inverter15/1
  Inverter17/1 -> OUT/1, Logical6/2
  Inverter16/1 -> Inverter17/1
  EN/1 -> Logical6/1
  Inverter15/1 -> Inverter16/1

== system TRNG_test01/Random Bit Gen.6/RO1 ==
  EN : Inport
  Inverter15 : xbsIndex_r4/Inverter  en=off  latency=1  dbl_ovrd=off  block_type=inv
  Inverter16 : xbsIndex_r4/Inverter  en=off  latency=1  dbl_ovrd=off  block_type=inv
  Inverter17 : xbsIndex_r4/Inverter  en=off  latency=1  dbl_ovrd=off  block_type=inv
  Logical6 : xbsIndex_r4/Logical  logical_function=AND  inputs=2  en=off  latency=1  precision=Full  arith_type=Unsigned  n_bits=16  bin_pt=0  align_bp=on  dbl_ovrd=off  block_type=logical
  OUT : Outport
  wires:
  Logical6/1 -> Inverter15/1
  Inverter17/1 -> OUT/1, Logical6/2
  Inverter16/1 -> Inverter17/1
  EN/1 -> Logical6/1
  Inverter15/1 -> Inverter16/1

== system TRNG_test01/Random Bit Gen.6/RO2 ==
  EN : Inport
  Inverter15 : xbsIndex_r4/Inverter  en=off  latency=1  dbl_ovrd=off  block_type=inv
  Inverter16 : xbsIndex_r4/Inverter  en=off  latency=1  dbl_ovrd=off  block_type=inv
  Inverter17 : xbsIndex_r4/Inverter  en=off  latency=1  dbl_ovrd=off  block_type=inv
  Logical6 : xbsIndex_r4/Logical  logical_function=AND  inputs=2  en=off  latency=1  precision=Full  arith_type=Unsigned  n_bits=16  bin_pt=0  align_bp=on  dbl_ovrd=off  block_type=logical
  OUT : Outport
  wires:
  Logical6/1 -> Inverter15/1
  Inverter17/1 -> OUT/1, Logical6/2
  Inverter16/1 -> Inverter17/1
  EN/1 -> Logical6/1
  Inverter15/1 -> Inverter16/1

== system TRNG_test01/Random Bit Gen.6/RO3 ==
  EN : Inport
  Inverter15 : xbsIndex_r4/Inverter  en=off  latency=1  dbl_ovrd=off  block_type=inv
  Inverter16 : xbsIndex_r4/Inverter  en=off  latency=1  dbl_ovrd=off  block_type=inv
  Inverter17 : xbsIndex_r4/Inverter  en=off  latency=1  dbl_ovrd=off  block_type=inv
  Logical6 : xbsIndex_r4/Logical  logical_function=AND  inputs=2  en=off  latency=1  precision=Full  arith_type=Unsigned  n_bits=16  bin_pt=0  align_bp=on  dbl_ovrd=off  block_type=logical
  OUT : Outport
  wires:
  Logical6/1 -> Inverter15/1
  Inverter17/1 -> OUT/1, Logical6/2
  Inverter16/1 -> Inverter17/1
  EN/1 -> Logical6/1
  Inverter15/1 -> Inverter16/1

== system TRNG_test01/Random Bit Gen.6/RO4 ==
  EN : Inport
  Inverter15 : xbsIndex_r4/Inverter  en=off  latency=1  dbl_ovrd=off  block_type=inv
  Inverter16 : xbsIndex_r4/Inverter  en=off  latency=1  dbl_ovrd=off  block_type=inv
  Inverter17 : xbsIndex_r4/Inverter  en=off  latency=1  dbl_ovrd=off  block_type=inv
  Logical6 : xbsIndex_r4/Logical  logical_function=AND  inputs=2  en=off  latency=1  precision=Full  arith_type=Unsigned  n_bits=16  bin_pt=0  align_bp=on  dbl_ovrd=off  block_type=logical
  OUT : Outport
  wires:
  Logical6/1 -> Inverter15/1
  Inverter17/1 -> OUT/1, Logical6/2
  Inverter16/1 -> Inverter17/1
  EN/1 -> Logical6/1
  Inverter15/1 -> Inverter16/1
